simulink model "RT_DT1_blocks"  (R2013a)
settings: Solver=ode45  StartTime=0.0  StopTime=10.0  RelTol=1e-3
values from neighbouring files (symbols this model uses):
  k = 1    [RT_Klausur_SS2014.m]    (also in RT_ctrl_analyse_proc.m = 5; RT_dennis_draussen.m = 50; RT_klausurvorb.m = 0.2; RT_lab_paramLead.m)
  sel = [1 2; 4 5; 7 8]    [RT_Klausur_SS2014.m]    (also in RT_ctrl_analyse_proc.m = 3; RT_gui_guide_2_b.m)
  T = 0.1    [RT_ctrl_analyse_proc.m]    (also in RT_lab_paramLead.m = 10; RT_lead_lag_uebung.m; regelungstechnik.m = 0.008; s_schrittantwort.m = round(10*Tsum/2)/10)
settings Model: Creator=mainster  LastModifiedBy=mainster
settings DebuggingCC: SolverPrmCheckMsg=none

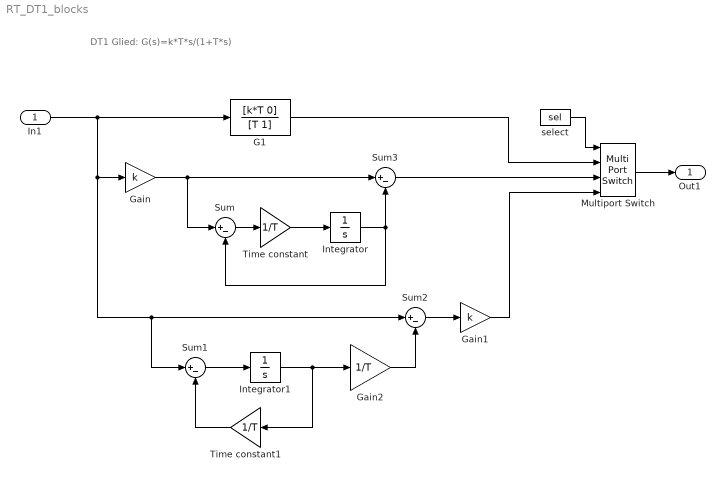
== system RT_DT1_blocks ==
  note: DT1 Glied: G(s)=k*T*s/(1+T*s)
  In1 : Inport
  G1 : TransferFcn  Numerator=[k*T 0]  Denominator=[T 1]
  Gain : Gain  Gain=k
  Gain1 : Gain  Gain=k
  Gain2 : Gain  Gain=1/T
  Integrator : Integrator
  Integrator1 : Integrator
  Multiport Switch : MultiPortSwitch
  Sum{,1..3} (4 alike) : Sum  Inputs=|+-
  Time constant : Gain  Gain=1/T
  Time constant1 : Gain  Gain=1/T
  select : Constant  Value=sel
  Out1 : Outport
  wires:
  Multiport Switch/1 -> Out1/1
  select/1 -> Multiport Switch/1
  G1/1 -> Multiport Switch/2
  Gain/1 -> Sum/1, Sum3/1
  Sum/1 -> Time constant/1
  Time constant/1 -> Integrator/1
  In1/1 -> Sum1/1, Sum2/1, Gain/1, G1/1
  Sum1/1 -> Integrator1/1
  Time constant1/1 -> Sum1/2
  Integrator1/1 -> Gain2/1, Time constant1/1
  Gain2/1 -> Sum2/2
  Sum2/1 -> Gain1/1
  Gain1/1 -> Multiport Switch/4
  Integrator/1 -> Sum3/2, Sum/2
  Sum3/1 -> Multiport Switch/3
